simulink model "BBK"  (Simulink 6.5)
settings: Solver=ode1  StartTime=0.0  StopTime=300  FixedStep=0.02  RelTol=1e-3
PostLoadFcn:
  | ,try, rti_mdl_postloadfcn(bdroot, 'UpdateModel', 280, 'rti1006'); catch, disp(lasterr); end,
settings Model: Creator=Cambustion  LastModifiedBy=Cambustion  BufferReuse=off  ProdHWDeviceType=Specified
settings OptimizationCC: BlockReduction=off  OptimizeBlockIOStorage=off  BufferReuse=off  ExpressionFolding=off  LocalBlockOutputs=off
settings HardwareCC: ProdIntDivRoundTo=Zero  ProdEndianess=LittleEndian  ProdHWDeviceType=Specified  TargetIntDivRoundTo=Zero  TargetEndianess=LittleEndian
settings RTWCC: SystemTargetFile=rti1006.tlc  MakeCommand=make_rti  TemplateMakefile=rti1006.tmf  Description=dSPACE DS1006 Hardware Platform  ProcessScript=rti1006_make_rtw_hook
settings STFCustomTargetCC: TargetFcnLib=ansi_tfl_tmw.mat  GenFloatMathFcnCalls=ANSI_C  ModelReferenceCompliant=off  MatFileLogging=on  SystemTargetFile=rti1006.tlc
settings GRTTargetCC: ModelReferenceCompliant=off  ExtModeMexFile=rti_comm_2
settings CustomProperty: DataType=RTWOptions_EnumType_C__dSpace_matlab_rti1006_tlc_rti1006_InitialSimState  Value=RUN
settings EnumStrPairs: String=RUN

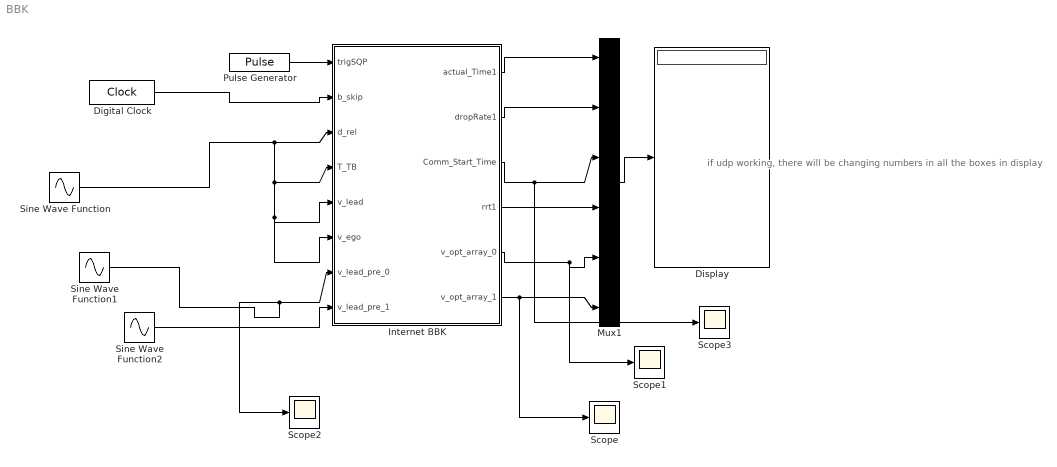
== system BBK ==
  note: if udp working, there will be changing
      |  numbers in all the boxes in display
  Digital Clock : DigitalClock  SampleTime=0.02
  Display : Display
  Internet BBK : Subsystem
  Mux1 : Mux  Inputs=[1 1 1 1 1 1]
  Pulse Generator : DiscretePulseGenerator  PulseType=Time based  Period=1  PulseWidth=20
  Scope{,1..3} (4 alike) : Scope
      Scope settings: TimeRange=10  YMin=37  YMax=40
      Scope2 settings: SaveName=ScopeData2
      Scope3 settings: TimeRange=10  SaveName=ScopeData3
  Sine Wave Function : Sin  SampleTime=0
  Sine Wave Function1 : Sin  Frequency=2  SampleTime=0
  Sine Wave Function2 : Sin  Frequency=4  SampleTime=0
  wires:
  Pulse Generator/1 -> Internet BBK/1(trigSQP)
  Sine Wave Function/1 -> Internet BBK/3(d_rel), Internet BBK/4(T_TB), Internet BBK/5(v_lead), Internet BBK/6(v_ego)
  Sine Wave Function1/1 -> Internet BBK/7(v_lead_pre_0), Scope2/1
  Sine Wave Function2/1 -> Internet BBK/8(v_lead_pre_1)
  Internet BBK/5(v_opt_array_0) -> Mux1/5, Scope1/1
  Internet BBK/4(rrt1) -> Mux1/4
  Internet BBK/3(Comm_Start_Time) -> Mux1/3, Scope3/1
  Internet BBK/2(dropRate1) -> Mux1/2
  Internet BBK/1(actual_Time1) -> Mux1/1
  Mux1/1 -> Display/1
  Internet BBK/6(v_opt_array_1) -> Mux1/6, Scope/1
  Digital Clock/1 -> Internet BBK/2(b_skip)

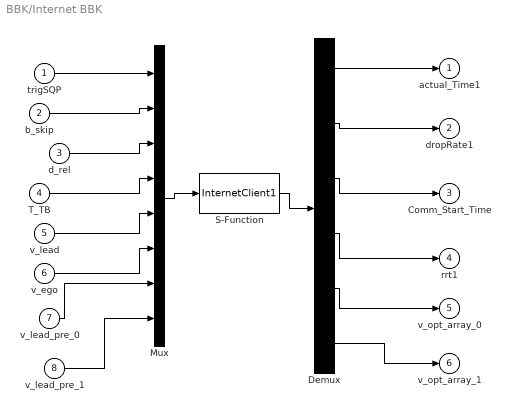
== system BBK/Internet BBK ==
  trigSQP : Inport  OutDataType=fixdt(1,16,0)  OutScaling=[]
  b_skip : Inport  Port=2  OutDataType=fixdt(1,16,0)  OutScaling=[]
  d_rel : Inport  Port=3  OutDataType=fixdt(1,16,0)  OutScaling=[]
  T_TB : Inport  Port=4  OutDataType=fixdt(1,16,0)  OutScaling=[]
  v_lead : Inport  Port=5  OutDataType=fixdt(1,16,0)  OutScaling=[]
  v_ego : Inport  Port=6  OutDataType=fixdt(1,16,0)  OutScaling=[]
  v_lead_pre_0 : Inport  Port=7  OutDataType=fixdt(1,16,0)  OutScaling=[]
  v_lead_pre_1 : Inport  Port=8  OutDataType=fixdt(1,16,0)  OutScaling=[]
  Demux : Demux  Outputs=[1 1 1 1 1 1]
  Mux : Mux  Inputs=8
  S-Function : S-Function  FunctionName=InternetClient1
  actual_Time1 : Outport  OutDataType=fixdt(1,16,0)  OutScaling=[]
  dropRate1 : Outport  Port=2  OutDataType=fixdt(1,16,0)  OutScaling=[]
  Comm_Start_Time : Outport  Port=3  OutDataType=fixdt(1,16,0)  OutScaling=[]
  rrt1 : Outport  Port=4  OutDataType=fixdt(1,16,0)  OutScaling=[]
  v_opt_array_0 : Outport  Port=5  OutDataType=fixdt(1,16,0)  OutScaling=[]
  v_opt_array_1 : Outport  Port=6  OutDataType=fixdt(1,16,0)  OutScaling=[]
  wires:
  trigSQP/1 -> Mux/1
  b_skip/1 -> Mux/2
  d_rel/1 -> Mux/3
  Demux/2 -> dropRate1/1
  Demux/4 -> rrt1/1
  Demux/1 -> actual_Time1/1
  Demux/5 -> v_opt_array_0/1
  Demux/3 -> Comm_Start_Time/1
  T_TB/1 -> Mux/4
  v_lead/1 -> Mux/5
  v_ego/1 -> Mux/6
  v_lead_pre_0/1 -> Mux/7
  v_lead_pre_1/1 -> Mux/8
  Demux/6 -> v_opt_array_1/1
  S-Function/1 -> Demux/1
  Mux/1 -> S-Function/1
